simulink model "crazyflie"  (R2023a)
settings: Solver=FixedStepDiscrete  StartTime=0.0  StopTime=160  FixedStep=0.001  RelTol=1e-3
settings Model: PauseTimes=7  Creator=Zrean  LastModifiedBy=bober
settings SolverCC: AlgebraicLoopSolver=TrustRegion
settings DataIOCC: ReturnWorkspaceOutputs=off
settings OptimizationCC: DefaultParameterBehavior=Inlined  UseDivisionForNetSlopeComputation=on  UseFloatMulNetSlope=on  UseSpecifiedMinMax=on  InlineInvariantSignals=on  PassReuseOutputArgsAs=Individual arguments  ZeroExternalMemoryAtStartup=off  ZeroInternalMemoryAtStartup=off  NoFixptDivByZeroProtection=on  EfficientFloat2IntCast=on  LifeSpan=1  EfficientTunableParamExpr=on
settings DebuggingCC: AlgebraicLoopMsg=error  ParameterTunabilityLossMsg=error  UnconnectedInputMsg=warning  UnconnectedOutputMsg=warning  UnconnectedLineMsg=warning  ArithmeticOperatorsInVariantConditions=warning
settings HardwareCC: ProdBitPerPointer=32  ProdBitPerSizeT=32  ProdBitPerPtrDiffT=32  ProdLargestAtomicInteger=Long  ProdLargestAtomicFloat=Double  ProdWordSize=32  ProdHWDeviceType=ARM Compatible->ARM Cortex
settings ModelReferenceCC: EnableRefExpFcnMdlSchedulingChecks=on
settings SFSimCC: SimUseLocalCustomCode=off  MATLABDynamicMemAlloc=off  CustomCodeUndefinedFunction=UseInterfaceOnly
settings RTWCC: Description=Embedded Coder  SystemTargetFile=ert.tlc  GenCodeOnly=on  TemplateMakefile=ert_default_tmf  GenerateReport=on  RTWUseLocalCustomCode=off  BuildConfiguration=Faster Runs  IncludeHyperlinkInReport=on  LaunchReport=on  GenerateTraceInfo=on  GenerateTraceReport=on  GenerateTraceReportSl=on  GenerateTraceReportSf=on  GenerateTraceReportEml=on  GenerateCodeMetricsReport=on
settings CodeAppCC: ForceParamTrailComments=on  IgnoreCustomStorageClasses=off  OperatorAnnotations=on  SimulinkDataObjDesc=on  SFDataObjDesc=on  MATLABFcnDesc=on  InsertBlockDesc=on  StateflowObjectComments=on  MATLABSourceComments=on
settings ERTTargetCC: TargetLangStandard=C99 (ISO)  MultiwordLength=2048  CombineSignalStateStructs=on  SuppressErrorStatus=on  SupportAbsoluteTime=off  SupportNonFinite=off  SupportComplex=off  InlinedParameterPlacement=NonHierarchical  ERTCustomFileTemplate=crazyflie_wrapper.tlc  ERTFilePackagingFormat=CompactWithDataFile
settings SimscapeCC: SimscapeNormalizeSystem=off

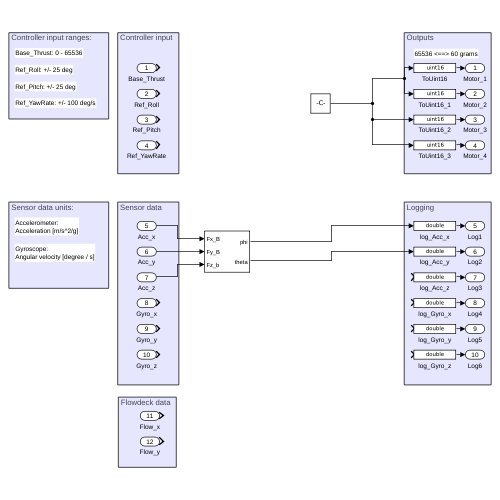
[thumbnail: Simulink's stored preview of the top-level diagram]
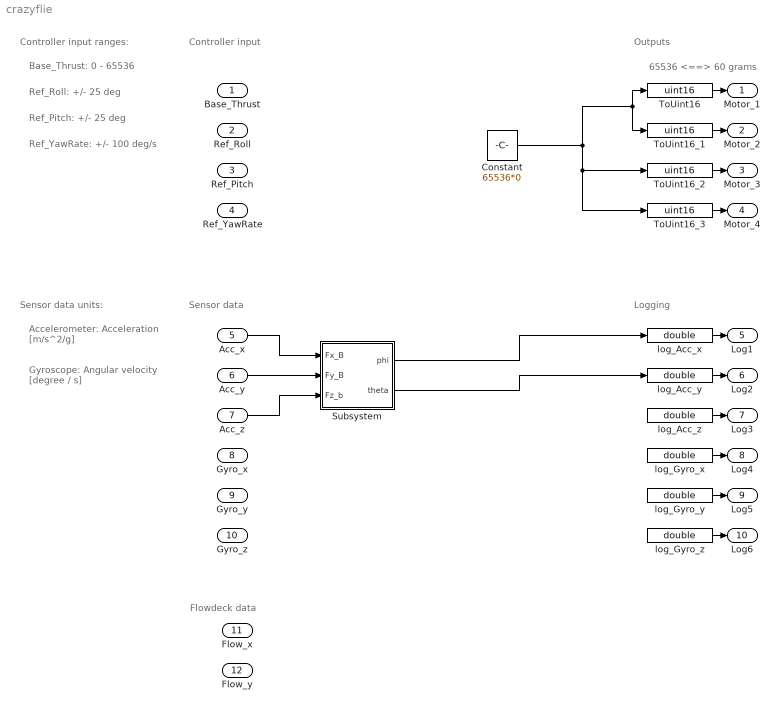
== system crazyflie ==
  note: 65536 <==> 60 grams
  note: Logging
  note: Outputs
  note: Sensor data
  note: Controller input
  note: Ref_Roll: +/- 25 deg
  note: Base_Thrust: 0 - 65536
  note: Ref_Pitch: +/- 25 deg
  note: Ref_YawRate: +/- 100 deg/s
  note: Controller input ranges:
  note: Gyroscope:
      | Angular velocity [degree / s]
  note: Accelerometer:
      | Acceleration [m/s^2/g]
  note: Sensor data units:
  note: Flowdeck data
  Base_Thrust : Inport  OutDataTypeStr=double
  Ref_Roll : Inport  Port=2  OutDataTypeStr=double
  Ref_Pitch : Inport  Port=3  OutDataTypeStr=double
  Ref_YawRate : Inport  Port=4  OutDataTypeStr=double
  Acc_x : Inport  Port=5  OutDataTypeStr=double  PortDimensions=1
  Acc_y : Inport  Port=6  OutDataTypeStr=double  PortDimensions=1
  Acc_z : Inport  Port=7  OutDataTypeStr=double  PortDimensions=1
  Gyro_x : Inport  Port=8  OutDataTypeStr=double  PortDimensions=1
  Gyro_y : Inport  Port=9  OutDataTypeStr=double  PortDimensions=1
  Gyro_z : Inport  Port=10  OutDataTypeStr=double  PortDimensions=1
  Flow_x : Inport  Port=11  OutDataTypeStr=int16  PortDimensions=1
  Flow_y : Inport  Port=12  OutDataTypeStr=int16  PortDimensions=1
  Constant : Constant  Value=65536*0
  Subsystem : Subsystem
  ToUint16 : DataTypeConversion  OutDataTypeStr=uint16  RndMeth=Floor
  ToUint16_1 : DataTypeConversion  OutDataTypeStr=uint16  RndMeth=Floor
  ToUint16_2 : DataTypeConversion  OutDataTypeStr=uint16  RndMeth=Floor
  ToUint16_3 : DataTypeConversion  OutDataTypeStr=uint16  RndMeth=Floor
  log_Acc_x : DataTypeConversion  OutDataTypeStr=double  RndMeth=Floor
  log_Acc_y : DataTypeConversion  OutDataTypeStr=double  RndMeth=Floor
  log_Acc_z : DataTypeConversion  OutDataTypeStr=double  RndMeth=Floor
  log_Gyro_x : DataTypeConversion  OutDataTypeStr=double  RndMeth=Floor
  log_Gyro_y : DataTypeConversion  OutDataTypeStr=double  RndMeth=Floor
  log_Gyro_z : DataTypeConversion  OutDataTypeStr=double  RndMeth=Floor
  Motor_1 : Outport  OutDataTypeStr=uint16  VectorParamsAs1DForOutWhenUnconnected=off  LockScale=on
  Motor_2 : Outport  Port=2  OutDataTypeStr=uint16  VectorParamsAs1DForOutWhenUnconnected=off  LockScale=on
  Motor_3 : Outport  Port=3  OutDataTypeStr=uint16  VectorParamsAs1DForOutWhenUnconnected=off  LockScale=on
  Motor_4 : Outport  Port=4  OutDataTypeStr=uint16  VectorParamsAs1DForOutWhenUnconnected=off  LockScale=on
  Log1 : Outport  Port=5  OutDataTypeStr=double  VectorParamsAs1DForOutWhenUnconnected=off
  Log2 : Outport  Port=6  OutDataTypeStr=double  VectorParamsAs1DForOutWhenUnconnected=off
  Log3 : Outport  Port=7  OutDataTypeStr=double  VectorParamsAs1DForOutWhenUnconnected=off
  Log4 : Outport  Port=8  OutDataTypeStr=double  VectorParamsAs1DForOutWhenUnconnected=off
  Log5 : Outport  Port=9  OutDataTypeStr=double  VectorParamsAs1DForOutWhenUnconnected=off
  Log6 : Outport  Port=10  OutDataTypeStr=double  VectorParamsAs1DForOutWhenUnconnected=off
  wires:
  ToUint16/1 -> Motor_1/1
  ToUint16_1/1 -> Motor_2/1
  ToUint16_2/1 -> Motor_3/1
  ToUint16_3/1 -> Motor_4/1
  log_Acc_x/1 -> Log1/1
  log_Acc_y/1 -> Log2/1
  log_Acc_z/1 -> Log3/1
  log_Gyro_x/1 -> Log4/1
  log_Gyro_y/1 -> Log5/1
  log_Gyro_z/1 -> Log6/1
  Constant/1 -> ToUint16_2/1, ToUint16_3/1, ToUint16/1, ToUint16_1/1
  Acc_x/1 -> Subsystem/1(Fx_B)
  Acc_y/1 -> Subsystem/2(Fy_B)
  Acc_z/1 -> Subsystem/3(Fz_b)
  Subsystem/1(phi) -> log_Acc_x/1
  Subsystem/2(theta) -> log_Acc_y/1

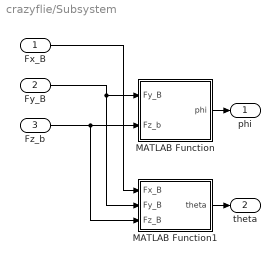
== system crazyflie/Subsystem ==
  Fx_B : Inport
  Fy_B : Inport  Port=2
  Fz_b : Inport  Port=3
  MATLAB Function : MATLAB Function  TreatAsAtomicUnit=on
  MATLAB Function1 : MATLAB Function  TreatAsAtomicUnit=on
  phi : Outport
  theta : Outport  Port=2
  wires:
  Fz_b/1 -> MATLAB Function1/3(Fz_B), MATLAB Function/2(Fz_b)
  MATLAB Function/1(phi) -> phi/1
  Fx_B/1 -> MATLAB Function1/1(Fx_B)
  Fy_B/1 -> MATLAB Function1/2(Fy_B), MATLAB Function/1(Fy_B)
  MATLAB Function1/1(theta) -> theta/1

== matlab function crazyflie/Subsystem/MATLAB Function ==
  data: Fy_B input; phi output; Fz_b input
function phi = fcn(Fy_B,Fz_b)

phi= arctan2(Fy_B,Fz_b);

== matlab function crazyflie/Subsystem/MATLAB Function1 ==
  data: Fx_B input; Fy_B input; theta output; Fz_B input
function theta = fcn(Fx_B,Fy_B,Fz_B)

theta = arctan2(-Fx_B,sqrt((Fy_B).^2+(Fz_B).^2));
